simulink model "IEEE_9bus_4"  (Simulink 8.4)
settings: Solver=ode4  StartTime=0.0  StopTime=inf  FixedStep=Ts  RelTol=1e-3
PostLoadFcn:
  | Ts=25e-6;Rs=5*1.867;cs=1.4080e-004;
InitFcn:
  | Ts=25e-6;Rs=5*1.867;cs=1.4080e-004;
undefined symbols (not defined in the file): another_event_name, gcbh, my_event_name, sps_rtmsupport
libraries: spsVIMeasurementModel x36, powerlib x34, powerlib_meascontrol x18, rtlab x4, artemis x3, sps_avr x3
(part 3 of 3)

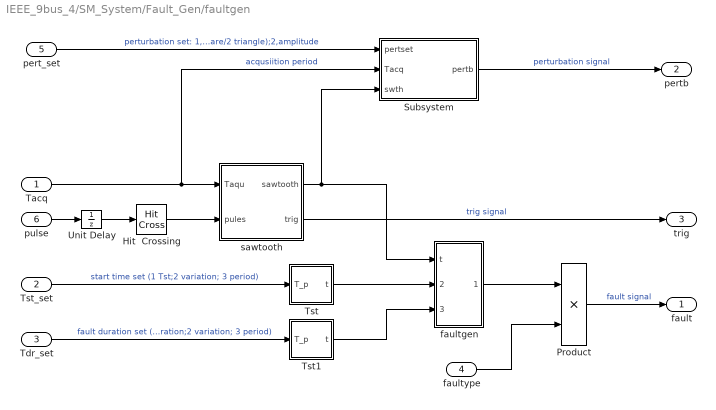
== system IEEE_9bus_4/SM_System/Fault_Gen/faultgen ==
  Tacq : Inport
  Tst_set : Inport  Port=2
  Tdr_set : Inport  Port=3
  faultype : Inport  Port=4
  pert_set : Inport  Port=5
  pulse : Inport  Port=6
  Hit  Crossing : HitCross  HitCrossingDirection=rising  SampleTime=Ts
  Product : Product  SampleTime=Ts  RndMeth=Zero
  Subsystem : Subsystem
  Tst : Subsystem
  Tst1 : Subsystem
  Unit Delay : UnitDelay  SampleTime=Ts
  faultgen : Subsystem
  sawtooth : Subsystem
  fault : Outport  SampleTime=Ts
  pertb : Outport  Port=2
  trig : Outport  Port=3
  wires:
  sawtooth/1(sawtooth) -> Subsystem/3(swth), faultgen/1(t)
  Tst/1(t) -> faultgen/2(Tstat)
  Tst1/1(t) -> faultgen/3(Tdur)
  Tacq/1 -> Subsystem/2(Tacq), sawtooth/1(Taqu)  "acqusiition period"
  pert_set/1 -> Subsystem/1(pertset)  "perturbation set: 1,(0 none/1 square/2 triangle);2,amplitude"
  Subsystem/1(pertb) -> pertb/1  "perturbation signal"
  sawtooth/2(trig) -> trig/1  "trig signal"
  Tst_set/1 -> Tst/1(T_p)  "start time set (1 Tst;2 variation; 3 period)"
  Tdr_set/1 -> Tst1/1(T_p)  "fault duration set (1 duration;2 variation; 3 period)"
  Hit  Crossing/1 -> sawtooth/2(pules)
  pulse/1 -> Unit Delay/1
  faultgen/1(fault) -> Product/1
  faultype/1 -> Product/2
  Product/1 -> fault/1  "fault signal"
  Unit Delay/1 -> Hit  Crossing/1

== system IEEE_9bus_4/SM_System/Generator BUS1x1/Subsystem1 ==
  In1 : Inport
  In2 : Inport  Port=2
  In3 : Inport  Port=3
  Gain : Gain  Gain=-1  SaturateOnIntegerOverflow=on  OutDataTypeStr=Inherit: Same as input  ParamDataTypeStr=Inherit: Same as input
  Mux : Mux  Inputs=2
  Selector : Selector  InputPortWidth=4  Indices=[4 3]
  Selector1 : Selector  InputPortWidth=4  Indices=[4 3]
  dw_123 : Outport
  T_23 : Outport  Port=2
  wires:
  Selector/1 -> Mux/2
  Mux/1 -> dw_123/1
  In1/1 -> Mux/1
  In2/1 -> Selector/1
  In3/1 -> Selector1/1
  Selector1/1 -> Gain/1
  Gain/1 -> T_23/1

== system IEEE_9bus_4/SM_System/Generator BUS2x1/Subsystem1 ==
  In1 : Inport
  In2 : Inport  Port=2
  In3 : Inport  Port=3
  Gain : Gain  Gain=-1  SaturateOnIntegerOverflow=on  OutDataTypeStr=Inherit: Same as input  ParamDataTypeStr=Inherit: Same as input
  Mux : Mux  Inputs=2
  Selector : Selector  InputPortWidth=4  Indices=[4 3]
  Selector1 : Selector  InputPortWidth=4  Indices=[4 3]
  dw_123 : Outport
  T_23 : Outport  Port=2
  wires:
  Selector/1 -> Mux/2
  Mux/1 -> dw_123/1
  In1/1 -> Mux/1
  In2/1 -> Selector/1
  In3/1 -> Selector1/1
  Selector1/1 -> Gain/1
  Gain/1 -> T_23/1

== system IEEE_9bus_4/SM_System/Generator BUS3x1/Subsystem1 ==
  In1 : Inport
  In2 : Inport  Port=2
  In3 : Inport  Port=3
  Gain : Gain  Gain=-1  SaturateOnIntegerOverflow=on  OutDataTypeStr=Inherit: Same as input  ParamDataTypeStr=Inherit: Same as input
  Mux : Mux  Inputs=2
  Selector : Selector  InputPortWidth=4  Indices=[4 3]
  Selector1 : Selector  InputPortWidth=4  Indices=[4 3]
  dw_123 : Outport
  T_23 : Outport  Port=2
  wires:
  Selector/1 -> Mux/2
  Mux/1 -> dw_123/1
  In1/1 -> Mux/1
  In2/1 -> Selector/1
  In3/1 -> Selector1/1
  Selector1/1 -> Gain/1
  Gain/1 -> T_23/1

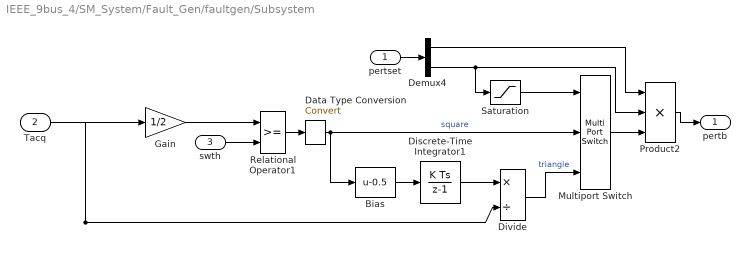
== system IEEE_9bus_4/SM_System/Fault_Gen/faultgen/Subsystem ==
  pertset : Inport
  Tacq : Inport  Port=2
  swth : Inport  Port=3
  Bias : Bias  Bias=-0.5
  Data Type Conversion : DataTypeConversion
  Demux4 : Demux  Outputs=2
  Discrete-Time Integrator1 : DiscreteIntegrator  gainval=2  SampleTime=Ts  LimitOutput=on  LowerSaturationLimit=0
  Divide : Product  Inputs=*/
  Gain : Gain  Gain=1/2
  Multiport Switch : MultiPortSwitch  Inputs=2
  Product2 : Product  Inputs=3  RndMeth=Zero
  Relational Operator1 : RelationalOperator  OutDataTypeStr=boolean
  Saturation : Saturate  UpperLimit=2  LowerLimit=1
  pertb : Outport
  wires:
  Gain/1 -> Relational Operator1/1
  Relational Operator1/1 -> Data Type Conversion/1
  Bias/1 -> Discrete-Time Integrator1/1
  Data Type Conversion/1 -> Bias/1, Multiport Switch/2  "square"
  Discrete-Time Integrator1/1 -> Divide/1
  Saturation/1 -> Multiport Switch/1
  Divide/1 -> Multiport Switch/3  "triangle"
  Multiport Switch/1 -> Product2/3
  Demux4/1 -> Product2/1
  Demux4/2 -> Saturation/1, Product2/2
  swth/1 -> Relational Operator1/2
  Tacq/1 -> Gain/1, Divide/2
  pertset/1 -> Demux4/1
  Product2/1 -> pertb/1

== system IEEE_9bus_4/SM_System/Fault_Gen/faultgen/Tst ==
  note: Prevents division by 0 at initial step
      | if a delay 1/Z is used before hand
  T_p : Inport
  Add : Sum
  Demux : Demux  Outputs=3
  Discrete-Time Integrtor : DiscreteIntegrator  ExternalReset=rising  SampleTime=-1
  Divide : Product  Inputs=*/
  Memory : Memory
  Relational Operator : RelationalOperator  OutDataTypeStr=boolean
  Saturation : Saturate  UpperLimit=inf  LowerLimit=0.0001
  t : Outport
  wires:
  Relational Operator/1 -> Discrete-Time Integrtor/2
  Memory/1 -> Relational Operator/1
  Discrete-Time Integrtor/1 -> Add/2, Memory/1
  Divide/1 -> Discrete-Time Integrtor/1
  T_p/1 -> Demux/1
  Demux/1 -> Add/1
  Demux/2 -> Divide/1, Relational Operator/2
  Add/1 -> t/1
  Demux/3 -> Saturation/1
  Saturation/1 -> Divide/2

== system IEEE_9bus_4/SM_System/Fault_Gen/faultgen/Tst1 ==
  note: Prevents division by 0 at initial step
      | if a delay 1/Z is used before hand
  T_p : Inport
  Add : Sum
  Demux : Demux  Outputs=3
  Discrete-Time Integrtor : DiscreteIntegrator  ExternalReset=rising  SampleTime=-1
  Divide : Product  Inputs=*/
  Memory : Memory
  Relational Operator : RelationalOperator  OutDataTypeStr=boolean
  Saturation : Saturate  UpperLimit=inf  LowerLimit=0.0001
  t : Outport
  wires:
  Relational Operator/1 -> Discrete-Time Integrtor/2
  Memory/1 -> Relational Operator/1
  Discrete-Time Integrtor/1 -> Add/2, Memory/1
  Divide/1 -> Discrete-Time Integrtor/1
  T_p/1 -> Demux/1
  Demux/1 -> Add/1
  Demux/2 -> Divide/1, Relational Operator/2
  Add/1 -> t/1
  Demux/3 -> Saturation/1
  Saturation/1 -> Divide/2

== system IEEE_9bus_4/SM_System/Fault_Gen/faultgen/faultgen ==
  t : Inport
  Tstat : Inport  Port=2
  Tdur : Inport  Port=3
  Add : Sum
  Logical Operator : Logic  AllPortsSameDT=off  OutDataTypeStr=boolean
  Relational Operator1 : RelationalOperator  Operator=<=  OutDataTypeStr=boolean
  Relational Operatr : RelationalOperator  OutDataTypeStr=boolean
  fault : Outport
  wires:
  Add/1 -> Relational Operator1/2
  Relational Operator1/1 -> Logical Operator/2
  Relational Operatr/1 -> Logical Operator/1
  t/1 -> Relational Operatr/1, Relational Operator1/1
  Logical Operator/1 -> fault/1
  Tdur/1 -> Add/2
  Tstat/1 -> Relational Operatr/2, Add/1

== system IEEE_9bus_4/SM_System/Fault_Gen/faultgen/sawtooth ==
  Taqu : Inport
  pules : Inport  Port=2
  Constant : Constant
  Data Type Conversion : DataTypeConversion
  Discrete-Time Integrator : DiscreteIntegrator  ExternalReset=rising  SampleTime=Ts
  Logical Operator : Logic  AllPortsSameDT=off
  Memory : Memory
  Relational Operator : RelationalOperator  OutDataTypeStr=boolean
  Voltage and Current Bus1 : Scope  NumInputPorts=2
      settings: TimeRange=1  YMin=0.0625~-1  YMax=0.1~1  SaveName=mach8  MaxDataPoints=15000
  sawtooth : Outport
  trig : Outport  Port=2
  wires:
  Constant/1 -> Discrete-Time Integrator/1
  Discrete-Time Integrator/1 -> Memory/1, sawtooth/1, Voltage and Current Bus1/1
  Memory/1 -> Relational Operator/1
  Logical Operator/1 -> Discrete-Time Integrator/2, Data Type Conversion/1
  Relational Operator/1 -> Logical Operator/2
  pules/1 -> Logical Operator/1
  Taqu/1 -> Relational Operator/2
  Data Type Conversion/1 -> trig/1
